simulink model "Lab2_First_Order"  (R2023a)
settings: Solver=VariableStepAuto  StartTime=0.0  StopTime=10.0  RelTol=1e-3
settings Model: Creator=Lenovo  LastModifiedBy=Lenovo

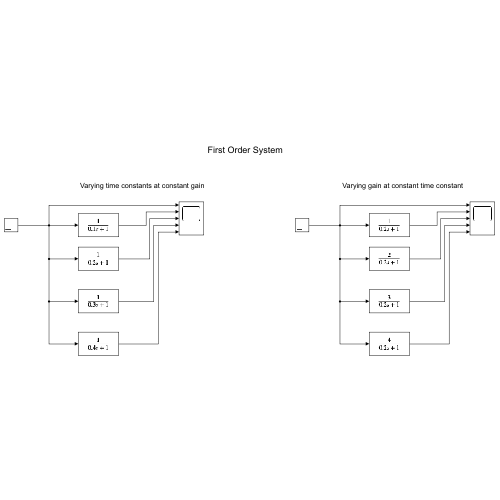
[thumbnail: Simulink's stored preview of the top-level diagram]
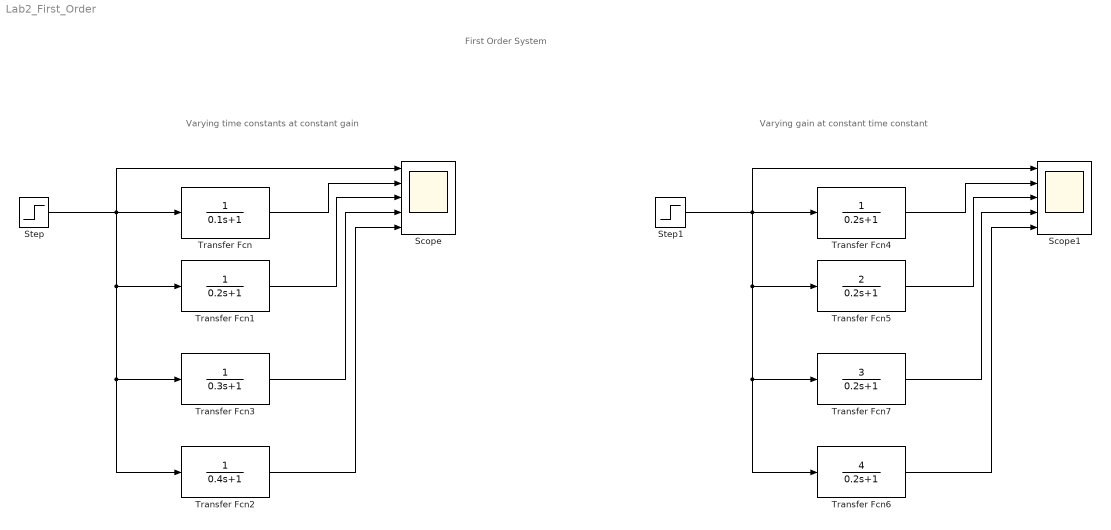
== system Lab2_First_Order ==
  note: First Order System
  note: Varying time constants at constant gain
  note: Varying gain at constant time constant
  Scope : Scope  NumInputPorts=5
  Scope1 : Scope  NumInputPorts=5
  Step : Step  SampleTime=0
  Step1 : Step  SampleTime=0
  Transfer Fcn : TransferFcn  Denominator=[0.1 1]
  Transfer Fcn1 : TransferFcn  Denominator=[0.2 1]
  Transfer Fcn2 : TransferFcn  Denominator=[0.4 1]
  Transfer Fcn3 : TransferFcn  Denominator=[0.3 1]
  Transfer Fcn4 : TransferFcn  Denominator=[0.2 1]
  Transfer Fcn5 : TransferFcn  Numerator=[2]  Denominator=[0.2 1]
  Transfer Fcn6 : TransferFcn  Numerator=[4]  Denominator=[0.2 1]
  Transfer Fcn7 : TransferFcn  Numerator=[3]  Denominator=[0.2 1]
  wires:
  Transfer Fcn/1 -> Scope/2
  Step/1 -> Transfer Fcn2/1, Transfer Fcn3/1, Transfer Fcn1/1, Scope/1, Transfer Fcn/1
  Transfer Fcn1/1 -> Scope/3
  Transfer Fcn3/1 -> Scope/4
  Transfer Fcn2/1 -> Scope/5
  Step1/1 -> Transfer Fcn6/1, Transfer Fcn7/1, Transfer Fcn5/1, Scope1/1, Transfer Fcn4/1
  Transfer Fcn7/1 -> Scope1/4
  Transfer Fcn6/1 -> Scope1/5
  Transfer Fcn5/1 -> Scope1/3
  Transfer Fcn4/1 -> Scope1/2
